simulink model "test_SOC_multi_cell"  (R2024a)
settings: Solver=FixedStepAuto  StartTime=0.0  StopTime=3600*24  FixedStep=1  RelTol=1e-3
libraries: simulink x3
settings Model: DataDictionary=SOXDictionaryGotion.sldd  Creator=mmackenzie  LastModifiedBy=mmackenzie
settings OptimizationCC: DefaultUnderspecifiedDataType=single
settings DebuggingCC: ParamPrecisionLossAbsoluteDiffThreshold=1e-10  ParamPrecisionLossRelativeDiffThreshold=1e-6  AllowSymbolicDim=off

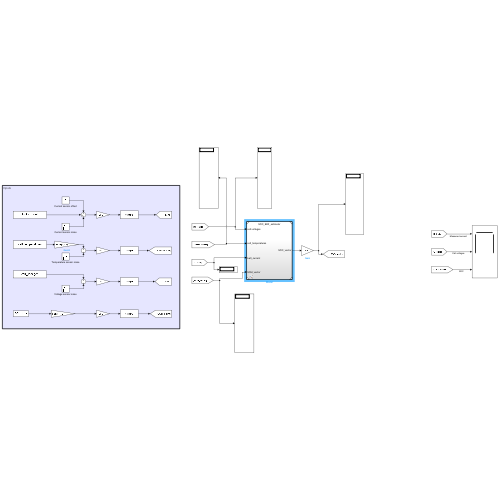
[thumbnail: Simulink's stored preview of the top-level diagram]
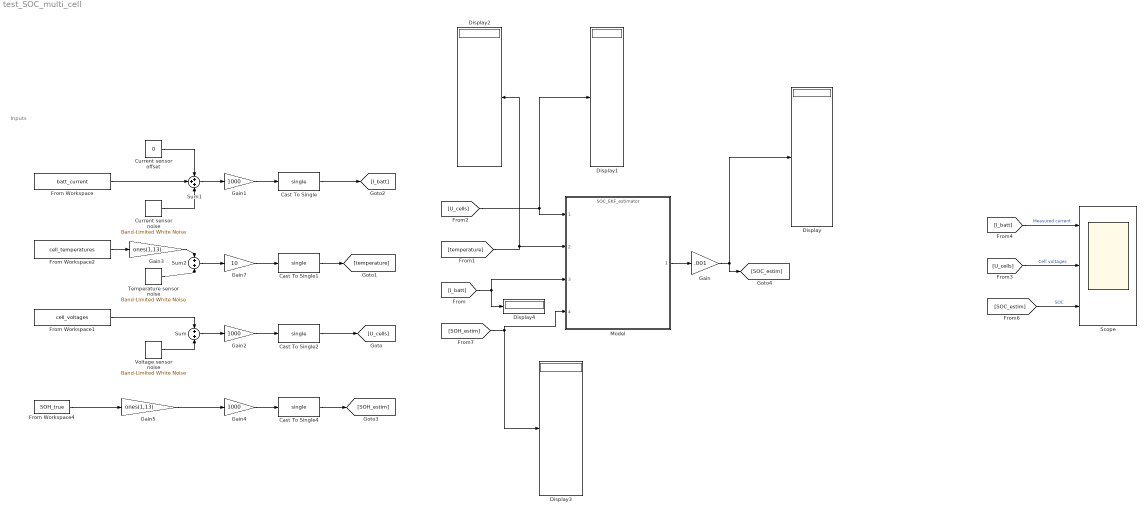
== system test_SOC_multi_cell ==
  note: Inputs
  Cast To Single{,1..2,4} (4 alike) : DataTypeConversion  OutDataTypeStr=single  SaturateOnIntegerOverflow=off  RndMeth=Floor
  Current sensor noise : simulink/Sources/Band-Limited White Noise  Cov=.1  Ts=1  seed=42
  Current sensor offset : Constant  Value=0
  Display{,1..4} (5 alike) : Display
  From Workspace : FromWorkspace  VariableName=batt_current
  From Workspace1 : FromWorkspace  VariableName=cell_voltages
  From Workspace2 : FromWorkspace  VariableName=cell_temperatures
  From Workspace4 : FromWorkspace  VariableName=SOH_true
  Gain : Gain  Gain=.001
  Gain1 : Gain  Gain=1000
  Gain2 : Gain  Gain=1000
  Gain3 : Gain  Gain=ones(1,13)
  Gain4 : Gain  Gain=1000
  Gain5 : Gain  Gain=ones(1,13)
  Gain7 : Gain  Gain=10
  Model : ModelReference  ModelNameDialog=SOC_EKF_estimator.slx  SimulationMode=Normal  ModelReferenceVersion=1.41
  Scope : Scope  NumInputPorts=3
  Sum : Sum
  Sum1 : Sum  Inputs=+++
  Sum2 : Sum
  Temperature sensor noise : simulink/Sources/Band-Limited White Noise  Cov=1  Ts=1  seed=42
  Voltage sensor noise : simulink/Sources/Band-Limited White Noise  Cov=1e-6  Ts=1  seed=42
  wires:
  [U_cells] -> Model/1, Display1/1
  [I_batt] -> Scope/1  "Measured current"
  Model/1 -> Gain/1
  [SOC_estim] -> Scope/3  "SOC"
  From Workspace2/1 -> Gain3/1
  From Workspace/1 -> Sum1/2
  Sum2/1 -> Gain7/1
  Current sensor offset/1 -> Sum1/1
  From Workspace1/1 -> Sum/1
  Sum/1 -> Gain2/1
  Temperature sensor noise/1 -> Sum2/2
  From Workspace4/1 -> Gain5/1
  Sum1/1 -> Gain1/1
  Current sensor noise/1 -> Sum1/3
  Voltage sensor noise/1 -> Sum/2
  [SOH_estim] -> Model/4, Display3/1
  [temperature] -> Model/2, Display2/1
  [I_batt] -> Model/3, Display4/1
  Gain/1 -> [SOC_estim], Display/1
  Gain1/1 -> Cast To Single/1
  Gain7/1 -> Cast To Single1/1
  Gain2/1 -> Cast To Single2/1
  Gain4/1 -> Cast To Single4/1
  Cast To Single/1 -> [I_batt]
  Cast To Single1/1 -> [temperature]
  Cast To Single2/1 -> [U_cells]
  Cast To Single4/1 -> [SOH_estim]
  [U_cells] -> Scope/2  "Cell voltages"
  Gain3/1 -> Sum2/1
  Gain5/1 -> Gain4/1
